simulink model "GVCU_HIL_simscape"  (R2026a)
settings: Solver=ode3  StartTime=0  StopTime=10  FixedStep=0.001
model workspace (MAT data in the model file):
  CANoelibParameters : object (value not decoded)
values from neighbouring files (symbols this model uses):
  acc_pedal_data = pedal_data.accelerator_pedal_position_t0    [Init_Simscape_main.m]
  acc_pedal_time = pedal_data.t0    [Init_Simscape_main.m]
  brk_pedal_data = brake_pedal_data.shared_brakes_drvrBrkPedlPerc_t0    [Init_Simscape_main.m]
  brk_pedal_time = brake_pedal_data.t0    [Init_Simscape_main.m]
  cycle_len = zeros(1, num_cycles)    [Init_Simscape_main.m]
  cycle_speed_matrix = zeros(max_cycle_len, num_cycles)    [Init_Simscape_main.m]
  cycle_time_matrix = zeros(max_cycle_len, num_cycles)    [Init_Simscape_main.m]
  veh_speed_data = speed_data.shared_dynamicsVso_vehVelLgt_t0    [Init_Simscape_main.m]
  veh_speed_time = speed_data.t0    [Init_Simscape_main.m]
undefined symbols (not defined in the file or in its folder): Active, aero, AuxActive, bat, brake, config, environment, FL, FL_prs_voltage, FR, FR_prs_voltage, front, pos, powertrain, rear, RL, RL_prs_voltage, RR, RR_prs_voltage, tir, veh, VGetRawValueFlag, Voltage, VT2816_1_Ch1, VT2816_1_Ch2, VT2816_1_Ch3, VT2816_1_Ch4, VT2816_3_Ch13, VT2816_3_Ch14, VT7101_1_Out2, VTS, X, Y, Z
libraries: sm_lib x358, fl_lib x272, nesl_utility x193, canoelib x127, sdl_lib x36, autolibsharedcoupling x21, autolibcoupling x9, slpidlib x7, simulink x3, autolibshareddiff x3, autolibshared x3, autolibutils x1
(part 17 of 17)

== system GVCU_HIL_simscape/vehicle/powertrain/motor/Subsystem ==
  EM_trq_out : Inport
  Ideal Torque Source1 : fl_lib/Mechanical/Mechanical Sources/Ideal Torque Source
  MRRef1 : fl_lib/Mechanical/Rotational Elements/Mechanical Rotational Reference
  PS Lookup Table (2D)1 : fl_lib/Physical Signals/Lookup Tables/PS Lookup Table (2D)  x1=[-1 powertrain.motor.throttle_bp]  x2=[flip(-powertrain.motor.rpm_bp(2:end)) powertrain.motor.rpm_bp] rad/s  f=[flip(-powertrain.motor.torque_bp(2:end)) -powertrain.motor.torque_bp; flip(powertrain.motor.torque_map(1,2:end)) powertrain.motor.torque_map(1,:); flip(powertrain.motor.torque_map(2,2:end)) powertrain.motor.torque_map(2,:)]  interp_method=simscape.enum.interpolation.linear  extrap_method=simscape.enum.extrapolation.nearest
  Simulink-PS Converter : nesl_utility/Simulink-PS Converter  Commented=on  PhysicalDomain=network_engine_domain  SubClassName=ps_input  LeftPortType=input  RightPortType=output  PseudoPeriodic=off  Frequencies=[]  NoiseDistribution=none  NoiseParameters=[]  Unit=1  AffineConversion=off  FilteringAndDerivatives=provide  SimscapeFilterOrder=1  InputFilterTimeConstant=0.001  UdotUserProvided=0
  throttle : PMIOPort  Side=Left
  omega : PMIOPort  Port=2  Side=Left
  Conn2 : PMIOPort  Port=3  Side=Right
  wires:
  EM_trq_out/1 -> Simulink-PS Converter/1
  connections:
  MRRef1/LConn1 -- Ideal Torque Source1/RConn2
  Ideal Torque Source1/LConn1 -- Conn2/RConn1
  PS Lookup Table (2D)1/LConn2 -- omega/RConn1
  throttle/RConn1 -- PS Lookup Table (2D)1/LConn1
  PS Lookup Table (2D)1/RConn1 -- Ideal Torque Source1/RConn1

== system GVCU_HIL_simscape/vehicle/powertrain/motor/Subsystem3 ==
  Ideal Rotational Motion Sensor : fl_lib/Mechanical/Mechanical Sensors/Ideal Rotational Motion Sensor  reference=foundation.enum.MeasurementReference.difference  acceleration_port=false  velocity_port=true  position_port=false  wrap_angle=false  offset=0 rad
  Ideal Torque Sensor : fl_lib/Mechanical/Mechanical Sensors/Ideal Torque Sensor
  Mechanical Rotational Reference : fl_lib/Mechanical/Rotational Elements/Mechanical Rotational Reference
  PS-Simulink Converter1 : nesl_utility/PS-Simulink Converter  PhysicalDomain=network_engine_domain  SubClassName=ps_output  LeftPortType=input  RightPortType=output  PseudoPeriodic=off  Frequencies=[]  VectorFormat=inherit  Unit=inherit  AffineConversion=off
  PS-Simulink Converter6 : nesl_utility/PS-Simulink Converter  PhysicalDomain=network_engine_domain  SubClassName=ps_output  LeftPortType=input  RightPortType=output  PseudoPeriodic=off  Frequencies=[]  VectorFormat=inherit  Unit=inherit  AffineConversion=off
  in : PMIOPort  Side=Left
  out : PMIOPort  Port=2  Side=Right
  w : Outport
  t : Outport  Port=2
  wires:
  PS-Simulink Converter6/1 -> w/1
  PS-Simulink Converter1/1 -> t/1
  connections:
  Mechanical Rotational Reference/LConn1 -- Ideal Rotational Motion Sensor/RConn1
  PS-Simulink Converter6/LConn1 -- Ideal Rotational Motion Sensor/RConn2
  PS-Simulink Converter1/LConn1 -- Ideal Torque Sensor/RConn2
  in/RConn1 -- Ideal Torque Sensor/LConn1 -- Ideal Rotational Motion Sensor/LConn1
  Ideal Torque Sensor/RConn1 -- out/RConn1

== system GVCU_HIL_simscape/vehicle/powertrain/motor/friction ==
  Ideal Rotational Motion Sensor : fl_lib/Mechanical/Mechanical Sensors/Ideal Rotational Motion Sensor  reference=foundation.enum.MeasurementReference.difference  acceleration_port=false  velocity_port=true  position_port=false  wrap_angle=false  offset=0 rad
  Inertia2 : fl_lib/Mechanical/Rotational Elements/Inertia  inertia=0.05 kg*m^2  num_ports=foundation.enum.numPorts2.one  w_specify=off  w_priority=High  w=0 rad/s  w_nominal_specify=off  w_nominal_value=1  w_nominal_unit=rad/s  t_specify=off  t_priority=None  t=0 N*m  t_nominal_specify=off  t_nominal_value=1  t_nominal_unit=N*m
  Mechanical Rotational Reference : fl_lib/Mechanical/Rotational Elements/Mechanical Rotational Reference
  PS Transfer Function : fl_lib/Physical Signals/Linear Operators/PS Transfer Function  transfer_function_type=foundation.enum.transfer_function_type.lag  T=0.01 s  T1=2 s  T2=1 s  reset_method=foundation.enum.IntegratorResetSpec.None  initial_condition_spec=foundation.enum.IntegratorICSpec.Internal  y0=0 rad/s
  in : PMIOPort  Side=Left
  out : PMIOPort  Port=2  Side=Right
  omega : PMIOPort  Port=3  Side=Right
  connections:
  in/RConn1 -- Inertia2/LConn1 -- Ideal Rotational Motion Sensor/LConn1 -- out/RConn1
  Ideal Rotational Motion Sensor/RConn2 -- PS Transfer Function/LConn1
  Mechanical Rotational Reference/LConn1 -- Ideal Rotational Motion Sensor/RConn1
  omega/RConn1 -- PS Transfer Function/RConn1

== system GVCU_HIL_simscape/vehicle/powertrain/motor/rev limiter ==
  <AccelCmd> : Inport
  PS Constant : fl_lib/Physical Signals/Sources/PS Constant  constant=10000*pi/30
  PS Divide : fl_lib/Physical Signals/Functions/PS Divide
  PS Lookup Table (1D) : fl_lib/Physical Signals/Lookup Tables/PS Lookup Table (1D)  x=[1 1.01] rad/s  f=[1 0]  interp_method=simscape.enum.interpolation.linear  extrap_method=simscape.enum.extrapolation.nearest
  PS Product : fl_lib/Physical Signals/Functions/PS Product
  Simulink-PS Converter : nesl_utility/Simulink-PS Converter  PhysicalDomain=network_engine_domain  SubClassName=ps_input  LeftPortType=input  RightPortType=output  PseudoPeriodic=off  Frequencies=[]  NoiseDistribution=none  NoiseParameters=[]  Unit=1  AffineConversion=off  FilteringAndDerivatives=filter  SimscapeFilterOrder=2  InputFilterTimeConstant=0.001  UdotUserProvided=0
  omega : PMIOPort  Side=Left
  throttle : PMIOPort  Port=2  Side=Right
  wires:
  <AccelCmd>/1 -> Simulink-PS Converter/1
  connections:
  PS Divide/LConn1 -- omega/RConn1
  PS Constant/RConn1 -- PS Divide/LConn2
  PS Divide/RConn1 -- PS Lookup Table (1D)/LConn1
  PS Product/LConn2 -- PS Lookup Table (1D)/RConn1
  Simulink-PS Converter/RConn1 -- PS Product/LConn1
  throttle/RConn1 -- PS Product/RConn1

== system GVCU_HIL_simscape/vehicle/powertrain/side gearbox/Subsystem1 ==
  Ideal Rotational Motion Sensor : fl_lib/Mechanical/Mechanical Sensors/Ideal Rotational Motion Sensor  reference=foundation.enum.MeasurementReference.difference  acceleration_port=false  velocity_port=true  position_port=false  wrap_angle=false  offset=0 rad
  Ideal Torque Sensor : fl_lib/Mechanical/Mechanical Sensors/Ideal Torque Sensor
  Mechanical Rotational Reference : fl_lib/Mechanical/Rotational Elements/Mechanical Rotational Reference
  PS-Simulink Converter1 : nesl_utility/PS-Simulink Converter  PhysicalDomain=network_engine_domain  SubClassName=ps_output  LeftPortType=input  RightPortType=output  PseudoPeriodic=off  Frequencies=[]  VectorFormat=inherit  Unit=inherit  AffineConversion=off
  PS-Simulink Converter6 : nesl_utility/PS-Simulink Converter  PhysicalDomain=network_engine_domain  SubClassName=ps_output  LeftPortType=input  RightPortType=output  PseudoPeriodic=off  Frequencies=[]  VectorFormat=inherit  Unit=inherit  AffineConversion=off
  in : PMIOPort  Side=Left
  out : PMIOPort  Port=2  Side=Right
  w : Outport
  t : Outport  Port=2
  wires:
  PS-Simulink Converter1/1 -> t/1
  PS-Simulink Converter6/1 -> w/1
  connections:
  Ideal Torque Sensor/RConn1 -- out/RConn1
  Ideal Rotational Motion Sensor/LConn1 -- Ideal Torque Sensor/LConn1 -- in/RConn1
  PS-Simulink Converter1/LConn1 -- Ideal Torque Sensor/RConn2
  PS-Simulink Converter6/LConn1 -- Ideal Rotational Motion Sensor/RConn2
  Mechanical Rotational Reference/LConn1 -- Ideal Rotational Motion Sensor/RConn1

== system GVCU_HIL_simscape/vehicle/powertrain/side gearbox/Subsystem3 ==
  Ideal Rotational Motion Sensor : fl_lib/Mechanical/Mechanical Sensors/Ideal Rotational Motion Sensor  reference=foundation.enum.MeasurementReference.difference  acceleration_port=false  velocity_port=true  position_port=false  wrap_angle=false  offset=0 rad
  Ideal Torque Sensor : fl_lib/Mechanical/Mechanical Sensors/Ideal Torque Sensor
  Mechanical Rotational Reference : fl_lib/Mechanical/Rotational Elements/Mechanical Rotational Reference
  PS-Simulink Converter1 : nesl_utility/PS-Simulink Converter  PhysicalDomain=network_engine_domain  SubClassName=ps_output  LeftPortType=input  RightPortType=output  PseudoPeriodic=off  Frequencies=[]  VectorFormat=inherit  Unit=inherit  AffineConversion=off
  PS-Simulink Converter6 : nesl_utility/PS-Simulink Converter  PhysicalDomain=network_engine_domain  SubClassName=ps_output  LeftPortType=input  RightPortType=output  PseudoPeriodic=off  Frequencies=[]  VectorFormat=inherit  Unit=inherit  AffineConversion=off
  in : PMIOPort  Side=Left
  out : PMIOPort  Port=2  Side=Right
  w : Outport
  t : Outport  Port=2
  wires:
  PS-Simulink Converter6/1 -> w/1
  PS-Simulink Converter1/1 -> t/1
  connections:
  Mechanical Rotational Reference/LConn1 -- Ideal Rotational Motion Sensor/RConn1
  PS-Simulink Converter6/LConn1 -- Ideal Rotational Motion Sensor/RConn2
  PS-Simulink Converter1/LConn1 -- Ideal Torque Sensor/RConn2
  in/RConn1 -- Ideal Torque Sensor/LConn1 -- Ideal Rotational Motion Sensor/LConn1
  Ideal Torque Sensor/RConn1 -- out/RConn1

== system GVCU_HIL_simscape/vehicle/powertrain/transmission/Subsystem3 ==
  Ideal Rotational Motion Sensor : fl_lib/Mechanical/Mechanical Sensors/Ideal Rotational Motion Sensor  reference=foundation.enum.MeasurementReference.difference  acceleration_port=false  velocity_port=true  position_port=false  wrap_angle=false  offset=0 rad
  Ideal Torque Sensor : fl_lib/Mechanical/Mechanical Sensors/Ideal Torque Sensor
  Mechanical Rotational Reference : fl_lib/Mechanical/Rotational Elements/Mechanical Rotational Reference
  PS-Simulink Converter1 : nesl_utility/PS-Simulink Converter  PhysicalDomain=network_engine_domain  SubClassName=ps_output  LeftPortType=input  RightPortType=output  PseudoPeriodic=off  Frequencies=[]  VectorFormat=inherit  Unit=inherit  AffineConversion=off
  PS-Simulink Converter6 : nesl_utility/PS-Simulink Converter  PhysicalDomain=network_engine_domain  SubClassName=ps_output  LeftPortType=input  RightPortType=output  PseudoPeriodic=off  Frequencies=[]  VectorFormat=inherit  Unit=inherit  AffineConversion=off
  in : PMIOPort  Side=Left
  out : PMIOPort  Port=2  Side=Right
  w : Outport
  t : Outport  Port=2
  wires:
  PS-Simulink Converter6/1 -> w/1
  PS-Simulink Converter1/1 -> t/1
  connections:
  Mechanical Rotational Reference/LConn1 -- Ideal Rotational Motion Sensor/RConn1
  PS-Simulink Converter6/LConn1 -- Ideal Rotational Motion Sensor/RConn2
  PS-Simulink Converter1/LConn1 -- Ideal Torque Sensor/RConn2
  in/RConn1 -- Ideal Torque Sensor/LConn1 -- Ideal Rotational Motion Sensor/LConn1
  Ideal Torque Sensor/RConn1 -- out/RConn1

== system GVCU_HIL_simscape/vehicle/powertrain/transmission/gear selector ==
  In1 : Inport
  Clutches Gear 1 : Constant  Value=[0 0 0 0 0 0 0 0 0]  SampleTime=0
  Clutches Gear 10 : Constant  Value=[0 0 0 0 0 0 0 1 0]  SampleTime=0
  Clutches Gear 11 : Constant  Value=[0 0 0 0 0 0 0 0 1]  SampleTime=0
  Clutches Gear 2 : Constant  Value=[1 0 0 0 0 0 0 0 0]  SampleTime=0
  Clutches Gear 3 : Constant  Value=[0 1 0 0 0 0 0 0 0]  SampleTime=0
  Clutches Gear 4 : Constant  Value=[0 0 0 0 0 0 0 0 0]  SampleTime=0
  Clutches Gear 5 : Constant  Value=[0 0 1 0 0 0 0 0 0]  SampleTime=0
  Clutches Gear 6 : Constant  Value=[0 0 0 1 0 0 0 0 0]  SampleTime=0
  Clutches Gear 7 : Constant  Value=[0 0 0 0 1 0 0 0 0]  SampleTime=0
  Clutches Gear 8 : Constant  Value=[0 0 0 0 0 1 0 0 0]  SampleTime=0
  Clutches Gear 9 : Constant  Value=[0 0 0 0 0 0 1 0 0]  SampleTime=0
  Demux : Demux  Outputs=9
  Multiport Switch : MultiPortSwitch  DataPortOrder=Specify indices  DataPortIndices={-1,0,1,2,3,4,5,6,7,8,9}  SaturateOnIntegerOverflow=off  InputSameDT=off
  Simulink-PS Converter{1..9} (9 alike) : nesl_utility/Simulink-PS Converter  PhysicalDomain=network_engine_domain  SubClassName=ps_input  LeftPortType=input  RightPortType=output  PseudoPeriodic=off  Frequencies=[]  NoiseDistribution=none  NoiseParameters=[]  Unit=1  AffineConversion=off  FilteringAndDerivatives=provide  SimscapeFilterOrder=1  InputFilterTimeConstant=0.001  UdotUserProvided=0
  1 : PMIOPort  Side=Right
  2 : PMIOPort  Port=2  Side=Right
  3 : PMIOPort  Port=3  Side=Right
  4 : PMIOPort  Port=4  Side=Right
  5 : PMIOPort  Port=5  Side=Right
  6 : PMIOPort  Port=6  Side=Right
  7 : PMIOPort  Port=7  Side=Right
  8 : PMIOPort  Port=8  Side=Right
  9 : PMIOPort  Port=9  Side=Right
  wires:
  Demux/5 -> Simulink-PS Converter4/1
  Clutches Gear 3/1 -> Multiport Switch/5
  Demux/4 -> Simulink-PS Converter3/1
  Clutches Gear 8/1 -> Multiport Switch/9
  Clutches Gear 5/1 -> Multiport Switch/6
  Clutches Gear 7/1 -> Multiport Switch/8
  Clutches Gear 10/1 -> Multiport Switch/11
  Clutches Gear 6/1 -> Multiport Switch/7
  Clutches Gear 11/1 -> Multiport Switch/12
  Clutches Gear 1/1 -> Multiport Switch/3
  Clutches Gear 2/1 -> Multiport Switch/4
  Demux/3 -> Simulink-PS Converter7/1
  Demux/7 -> Simulink-PS Converter6/1
  Demux/2 -> Simulink-PS Converter1/1
  Demux/1 -> Simulink-PS Converter2/1
  Clutches Gear 4/1 -> Multiport Switch/2
  Demux/8 -> Simulink-PS Converter8/1
  Demux/9 -> Simulink-PS Converter9/1
  Clutches Gear 9/1 -> Multiport Switch/10
  Multiport Switch/1 -> Demux/1
  Demux/6 -> Simulink-PS Converter5/1
  In1/1 -> Multiport Switch/1
  connections:
  Simulink-PS Converter2/RConn1 -- 1/RConn1
  3/RConn1 -- Simulink-PS Converter7/RConn1
  6/RConn1 -- Simulink-PS Converter5/RConn1
  4/RConn1 -- Simulink-PS Converter3/RConn1
  7/RConn1 -- Simulink-PS Converter6/RConn1
  5/RConn1 -- Simulink-PS Converter4/RConn1
  9/RConn1 -- Simulink-PS Converter9/RConn1
  8/RConn1 -- Simulink-PS Converter8/RConn1
  2/RConn1 -- Simulink-PS Converter1/RConn1

== system GVCU_HIL_simscape/vehicle/multibody/chassis/Subsystem/Subsystem ==
  1 : Inport
  2 : Inport  Port=2
  Add : Sum  Inputs=+++
  Constant : Constant  Value=eps
  Divide : Product  Inputs=*/
  Out1 : Outport
  wires:
  Divide/1 -> Out1/1
  Add/1 -> Divide/2
  2/1 -> Add/2
  1/1 -> Divide/1, Add/1
  Constant/1 -> Add/3

== system GVCU_HIL_simscape/vehicle/multibody/chassis/Subsystem/drag force ==
  PS Constant : fl_lib/Physical Signals/Sources/PS Constant  constant=1/2
  PS Constant1 : fl_lib/Physical Signals/Sources/PS Constant  constant=1.225 kg/m^3
  PS Constant2 : fl_lib/Physical Signals/Sources/PS Constant  constant=aero.A m^2
  PS Gain : fl_lib/Physical Signals/Functions/PS Gain  gain=-1
  PS Lookup Table (2D) : fl_lib/Physical Signals/Lookup Tables/PS Lookup Table (2D)  x1=aero.FRH m  x2=aero.RRH m  f=aero.Cd  interp_method=simscape.enum.interpolation.linear  extrap_method=simscape.enum.extrapolation.linear
  PS Product{,1..5} (6 alike) : fl_lib/Physical Signals/Functions/PS Product
  PS Sign : fl_lib/Physical Signals/Nonlinear Operators/PS Sign
  vx : PMIOPort  Side=Left
  fx : PMIOPort  Port=2  Side=Right
  frh : PMIOPort  Port=3  Side=Left
  rrh : PMIOPort  Port=4  Side=Left
  connections:
  vx/RConn1 -- PS Sign/LConn1 -- PS Product4/LConn2 -- PS Product4/LConn1
  PS Lookup Table (2D)/RConn1 -- PS Product/LConn2
  PS Product2/RConn1 -- PS Product1/LConn1
  PS Product3/RConn1 -- PS Product2/LConn1
  PS Constant1/RConn1 -- PS Product2/LConn2
  PS Constant2/RConn1 -- PS Product1/LConn2
  PS Product3/LConn2 -- PS Constant/RConn1
  PS Product4/RConn1 -- PS Product5/LConn1
  PS Product1/RConn1 -- PS Product/LConn1
  PS Gain/LConn1 -- PS Product/RConn1
  PS Product5/RConn1 -- PS Product3/LConn1
  PS Sign/RConn1 -- PS Product5/LConn2
  fx/RConn1 -- PS Gain/RConn1
  frh/RConn1 -- PS Lookup Table (2D)/LConn1
  rrh/RConn1 -- PS Lookup Table (2D)/LConn2

== system GVCU_HIL_simscape/vehicle/multibody/chassis/Subsystem/front downforce ==
  PS Constant : fl_lib/Physical Signals/Sources/PS Constant  constant=1/2
  PS Constant1 : fl_lib/Physical Signals/Sources/PS Constant  constant=1.225 kg/m^3
  PS Constant2 : fl_lib/Physical Signals/Sources/PS Constant  constant=aero.A m^2
  PS Lookup Table (2D) : fl_lib/Physical Signals/Lookup Tables/PS Lookup Table (2D)  x1=aero.FRH m  x2=aero.RRH m  f=aero.Clf  interp_method=simscape.enum.interpolation.linear  extrap_method=simscape.enum.extrapolation.linear
  PS Product{,1..4} (5 alike) : fl_lib/Physical Signals/Functions/PS Product
  vx : PMIOPort  Side=Left
  frh : PMIOPort  Port=2  Side=Left
  rrh : PMIOPort  Port=3  Side=Left
  fz : PMIOPort  Port=4  Side=Right
  connections:
  PS Product4/LConn2 -- PS Product4/LConn1 -- vx/RConn1
  PS Product2/LConn1 -- PS Product3/RConn1
  PS Product3/LConn2 -- PS Constant/RConn1
  PS Product2/RConn1 -- PS Product1/LConn1
  PS Product/LConn1 -- PS Product1/RConn1
  fz/RConn1 -- PS Product/RConn1
  PS Constant1/RConn1 -- PS Product2/LConn2
  PS Lookup Table (2D)/RConn1 -- PS Product/LConn2
  PS Product4/RConn1 -- PS Product3/LConn1
  PS Constant2/RConn1 -- PS Product1/LConn2
  PS Lookup Table (2D)/LConn1 -- frh/RConn1
  rrh/RConn1 -- PS Lookup Table (2D)/LConn2

== system GVCU_HIL_simscape/vehicle/multibody/chassis/Subsystem/rear downforce ==
  PS Constant : fl_lib/Physical Signals/Sources/PS Constant  constant=1/2
  PS Constant1 : fl_lib/Physical Signals/Sources/PS Constant  constant=1.225 kg/m^3
  PS Constant2 : fl_lib/Physical Signals/Sources/PS Constant  constant=aero.A m^2
  PS Lookup Table (2D) : fl_lib/Physical Signals/Lookup Tables/PS Lookup Table (2D)  x1=aero.FRH m  x2=aero.RRH m  f=aero.Clr  interp_method=simscape.enum.interpolation.linear  extrap_method=simscape.enum.extrapolation.linear
  PS Product{,1..4} (5 alike) : fl_lib/Physical Signals/Functions/PS Product
  vx : PMIOPort  Side=Left
  fz : PMIOPort  Port=2  Side=Right
  frh : PMIOPort  Port=3  Side=Left
  rrh : PMIOPort  Port=4  Side=Left
  connections:
  vx/RConn1 -- PS Product4/LConn2 -- PS Product4/LConn1
  PS Product3/LConn2 -- PS Constant/RConn1
  fz/RConn1 -- PS Product/RConn1
  PS Product4/RConn1 -- PS Product3/LConn1
  PS Lookup Table (2D)/RConn1 -- PS Product/LConn2
  PS Product/LConn1 -- PS Product1/RConn1
  PS Constant2/RConn1 -- PS Product1/LConn2
  PS Constant1/RConn1 -- PS Product2/LConn2
  PS Product2/RConn1 -- PS Product1/LConn1
  PS Product2/LConn1 -- PS Product3/RConn1
  frh/RConn1 -- PS Lookup Table (2D)/LConn1
  rrh/RConn1 -- PS Lookup Table (2D)/LConn2

== system GVCU_HIL_simscape/vehicle/multibody/chassis/Subsystem1/Subsystem ==
  note: not possible to handle pitch +/- 90 degrees according to source
  R : Inport
  Asin : Trigonometry  Operator=asin
  Atan1 : Trigonometry  Operator=atan2
  Atan2 : Trigonometry  Operator=atan2
  Demux : Demux  Outputs=2
  Demux1 : Demux  Outputs=2
  Gain : Gain  Gain=-1
  "R(3, 1)" : Selector  NumberOfDimensions=2  InputPortWidth=3  IndexOptions=Index vector (dialog),Index vector (dialog)  Indices=3,1  OutputSizes=1,1
  "R(3, 2:3)" : Selector  NumberOfDimensions=2  InputPortWidth=3  IndexOptions=Index vector (dialog),Index vector (dialog)  Indices=3,[2 3]  OutputSizes=1,1
  "R([2 1], 1)" : Selector  NumberOfDimensions=2  InputPortWidth=3  IndexOptions=Index vector (dialog),Index vector (dialog)  Indices=[2 1],1  OutputSizes=1,1
  Reshape : Reshape
  Reshape1 : Reshape
  Reshape2 : Reshape  OutputDimensionality=Customize  OutputDimensions=1
  roll : Outport  VectorParamsAs1DForOutWhenUnconnected=off
  pitch : Outport  Port=2  VectorParamsAs1DForOutWhenUnconnected=off
  yaw : Outport  Port=3  VectorParamsAs1DForOutWhenUnconnected=off
  wires:
  Demux/1 -> Atan2/1
  Atan2/1 -> Reshape2/1
  Demux1/1 -> Atan1/1
  Demux1/2 -> Atan1/2
  Gain/1 -> Asin/1
  Demux/2 -> Atan2/2
  "R([2 1], 1)"/1 -> Demux1/1
  Asin/1 -> Reshape1/1
  "R(3, 2:3)"/1 -> Demux/1
  Reshape/1 -> yaw/1
  Atan1/1 -> Reshape/1
  R/1 -> "R([2 1], 1)"/1, "R(3, 2:3)"/1, "R(3, 1)"/1
  Reshape2/1 -> roll/1
  Reshape1/1 -> pitch/1
  "R(3, 1)"/1 -> Gain/1

== system GVCU_HIL_simscape/vehicle/multibody/chassis/local coordinates/Subsystem ==
  In1 : Inport
  Asin : Trigonometry  Operator=asin
  Cos : Trigonometry  Operator=cos
  Demux : Demux  Outputs=3
  Derivative : Derivative
  Derivative1 : Derivative
  Divide : Product  Inputs=*/
  Divide1 : Product  Inputs=*/
  Gain : Gain  Gain=-1
  Mux : Mux  Inputs=2
  Selector : Selector  NumberOfDimensions=2  InputPortWidth=3  IndexOptions=Index vector (dialog),Index vector (dialog)  Indices=[1 2 3],2  OutputSizes=1,1
  Selector1 : Selector  NumberOfDimensions=2  InputPortWidth=3  IndexOptions=Index vector (dialog),Index vector (dialog)  Indices=[1 2 3],1  OutputSizes=1,1
  Selector2 : Selector  InputPortWidth=3  IndexOptions=Index vector (dialog)  Indices=[3]  OutputSizes=1
  Trigonometric Function1 : Trigonometry  Operator=atan2
  magnitude : Fcn  Expr=sqrt(u(1)*u(1)+u(2)*u(2))
  magnitude1 : Fcn  Expr=sqrt(u(1)*u(1)+u(2)*u(2)+u(3)*u(3))
  aRoll : Outport
  aPitch : Outport  Port=2
  nRoll : Outport  Port=3
  nPitch : Outport  Port=4
  wires:
  Derivative1/1 -> nRoll/1
  Derivative/1 -> nPitch/1
  Gain/1 -> aPitch/1, Derivative/1
  Selector2/1 -> Divide/1
  Asin/1 -> Gain/1
  magnitude1/1 -> Divide1/2
  Divide/1 -> Divide1/1
  Selector1/1 -> magnitude1/1, Selector2/1
  Cos/1 -> Divide/2
  Trigonometric Function1/1 -> Cos/1, aRoll/1, Derivative1/1
  Divide1/1 -> Asin/1
  Selector/1 -> Demux/1
  Demux/3 -> Trigonometric Function1/1
  Mux/1 -> magnitude/1
  Demux/1 -> Mux/1
  magnitude/1 -> Trigonometric Function1/2
  Demux/2 -> Mux/2
  In1/1 -> Selector/1, Selector1/1

== matlab function GVCU_HIL_simscape/Clutch handling/Offset_substraction/MATLAB Function ==
  data: drvMode input; y output; pPa input
function y = fcn(drvMode, pPa)
% drvMode : drive mode input
% pPa     : measured pressure input in Pa
% y       : pressure output with learned offset removed, in Pa

persistent prevDrvMode state timer sumP sampleCount offset

if isempty(prevDrvMode)
    prevDrvMode = drvMode;
    state = uint8(0);      % 0=idle, 1=wait, 2=average, 3=hold
    timer = 0.0;
    sumP = 0.0;
    sampleCount = uint32(0);
    offset = 0.0;
end

T = 0.0002;          % sample time [s]
WAIT_TIME = 0.5;     % wait time after drvMode becomes 1 [s]
AVG_TIME  = 0.2;     % averaging time [s]
ONE_BAR_PA = 1e5;    % 1 bar in Pa

% Trigger when drvMode becomes 1, regardless of previous value
if (prevDrvMode ~= 1) && (drvMode == 1)
    state = uint8(1);
    timer = 0.0;
    sumP = 0.0;
    sampleCount = uint32(0);
end

switch state
    case 0
        % Idle state

    case 1
        % Wait for 0.5 s
        timer = timer + T;
        if timer >= WAIT_TIME
            state = uint8(2);
            timer = 0.0;
            sumP = 0.0;
            sampleCount = uint32(0);
        end

    case 2
        % Average pressure for 0.2 s
        timer = timer + T;
        sumP = sumP + pPa;
        sampleCount = sampleCount + 1;

        if timer >= AVG_TIME
            if sampleCount > 0
                offset = sumP / double(sampleCount) - ONE_BAR_PA;
            else
                offset = 0.0;
            end
            state = uint8(3);
        end

    case 3
        % Hold learned offset
end

% Output compensated pressure
y = pPa - offset;

prevDrvMode = drvMode;

== matlab function GVCU_HIL_simscape/Powertrain (EV)/PID Speed Ctrl Mode/MATLAB Function1 ==
  settings: updateMethod=DISCRETE
  data: spdErr_rads input; trq_cmd output; trq_fwd input; trq_act input; lim_pos input; lim_neg input; reset input
function trq_cmd = speedPID(spdErr_rads, trq_fwd, trq_act, lim_pos, lim_neg, reset)
%#codegen
% Speed PID + feedforward, output clamped.
% Replicates inverter torque_handler.c trqHandlerSpeedCtrl()
%
% Inputs:
%   spdErr_rads  [rad/s]   speed error (spd_req - spd_fb), computed externally
%   trq_fwd      [Nm]      feedforward torque = GVCU torque request (added internally)
%   trq_act      [Nm]      actual motor torque feedback (e.g. EM_trq from motor model)
%   lim_pos      [Nm]      upper output clamp
%   lim_neg      [Nm]      lower output clamp
%   reset                  from spdCtrlReset block (>0.5 = active)
%
% Output:
%   trq_cmd  [Nm]      clamped torque command (PID + feedforward)
%
% Gains (caldata.c index 0, RPM-based, Ts=500us):
%   kp=2.5, ki=0.004, kaw=0.0035, kd=0

persistent intgl trqReqPrev

if isempty(intgl)
    intgl      = 0;
    trqReqPrev = 0;
end

Ts      = 0.0002;       % actual Simulink step size
Ts_inv  = 0.0005;       % inverter design step size
scale   = Ts / Ts_inv;  % = 0.4

% values from Set 3 
kp  = 2; %0.78;
ki  = 0.035 * scale;    % = 0.0016
kaw = 0.005 * scale;   % = 0.0014

if reset > 0.5
    intgl      = 0;
    trqReqPrev = 0;
    trq_cmd    = 0;
    return;
end

% Speed error in RPM (matches inverter: spdErr = spdReq - ctrlOutSpeed)
spdErr = spdErr_rads * (60 / (2*pi));

% Integrator update with anti-windup
% Matches inverter: spdIntgl += ki*spdErr + kaw*(trqAct - trqReq_prev_unclamped)
intgl = intgl + ki * spdErr + kaw * (trq_act - trqReqPrev);

% Unclamped total output (PID + feedforward)
trq_req_unc = kp * spdErr + intgl + trq_fwd;

% Clamp output
trq_cmd = max(lim_neg, min(lim_pos, trq_req_unc));

% Store unclamped total for next step's anti-windup
trqReqPrev = trq_cmd;

== matlab function GVCU_HIL_simscape/vehicle/powertrain/brakes/ABS/MATLAB Function ==
  data: decel input; ABSCmd input; decel_FL output; FL input; FR input; RL input; RR input; decel_FR output; decel_RL output; decel_RR output
function [decel_FL,decel_FR,decel_RL,decel_RR] = fcn(decel,ABSCmd,FL,FR,RL,RR)

if ABSCmd == 1
    decel_FL = decel*FL;
    decel_FR = decel*FR;
    decel_RL = decel*RL;
    decel_RR = decel*RR;
else
    decel_FL = decel;
    decel_FR = decel;
    decel_RL = decel;
    decel_RR = decel;
end

== matlab function GVCU_HIL_simscape/vehicle/powertrain/engine/TC/MATLAB Function ==
  data: accel input; accel_out output; TC input; slip_error input; TCCmd input
function accel_out = fcn(accel,TC,slip_error,TCCmd)

if TCCmd == 1 && slip_error > 0.1
    accel_out = accel*TC;
else
    accel_out = accel;
end

== matlab function GVCU_HIL_simscape/Driver/brake balance/brake balance ==
  data: right1 input; left1 input; BrakeBalCmd output; right2 input; left2 input; BrakeBal_max input; BrakeBal_min input; BrakeBal_default input; BrakeBal_act input
function BrakeBalCmd = fcn(right1,left1,right2,left2,BrakeBal_max,BrakeBal_min,BrakeBal_default,BrakeBal_act)

if BrakeBal_act == 0
    BrakeBal_act = BrakeBal_default;
end

if right1 == 1 && right2 == 0 && BrakeBal_act <= BrakeBal_max
    BrakeBal_act = BrakeBal_act + 0.01;
elseif left1 == 1 && left2 == 0 && BrakeBal_act >= BrakeBal_min
    BrakeBal_act = BrakeBal_act - 0.01;
end

BrakeBalCmd = BrakeBal_act;

== matlab function GVCU_HIL_simscape/Powertrain (EV)/PID Speed Controller/MATLAB Function ==
  settings: updateMethod=DISCRETE
  data: EM_Spd input; reset_out output; speed_req input; t input
function reset_out = spdCtrlReset(EM_Spd, speed_req, t)
% Resets PID integrator when both speeds are below threshold for 500ms.
% Matches real inverter: cInvStopSpeed = 20 RPM, SPD_CTRL_RESET_DELAY = 500ms
% Input t: simulation time from Clock block [s]

persistent stop_ts fired

if isempty(stop_ts)
    stop_ts = 0;
    fired   = false;
end

SPD_THRESHOLD  = 2.094;  % 20 RPM in rad/s  (= cInvStopSpeed)
RESET_DELAY_S  = 0.5;    % 500ms in s       (= SPD_CTRL_RESET_DELAY)

if (abs(EM_Spd) < SPD_THRESHOLD) && (abs(speed_req) < SPD_THRESHOLD)
    if stop_ts == 0
        stop_ts = t;     % Start timer: record entry time
    end

    if ((t - stop_ts) >= RESET_DELAY_S) && (~fired)
        reset_out = 1.0; % Rising edge -> reset PID integrator
        fired     = true;
    else
        reset_out = 0.0;
    end
else
    stop_ts   = 0;       % Reset timer
    fired     = false;   % Allow trigger again next standstill
    reset_out = 0.0;
end

== matlab function GVCU_HIL_simscape/Driver/gear/MATLAB Function ==
  settings: updateMethod=DISCRETE
  data: nEngine input; GearCmd output; ax input; gear_max input; nEngine_max input; nEngine_min input; t input; shift_delay input; gear_act input
function GearCmd = fcn(nEngine,ax,gear_max,nEngine_max,nEngine_min,t,shift_delay,gear_act)

if gear_act == 0
    gear_act = 1;
end

persistent last_time

if isempty(last_time)
    last_time = -inf;
end

if t - last_time >= shift_delay
    if nEngine > nEngine_max*pi/30 && gear_act < gear_max
        gear_act = gear_act + 1;
    end
    
    if nEngine < nEngine_min*pi/30 && gear_act > 1 && ax < 0
        gear_act = gear_act - 1;
    end
    last_time = t;
end

GearCmd = gear_act;

== matlab function GVCU_HIL_simscape/Inverter/INV ==
  data: inv_st_prev input; inv_st output; inv_ena_req input; motor_ena_req input; inv_shutdown_req input
function inv_st = fcn(inv_st_prev, inv_ena_req, motor_ena_req, inv_shutdown_req)
	switch inv_st_prev
		case 0
			if (1 == inv_ena_req)
				inv_st_local = 1;
			else
				inv_st_local = 0;
			end
		case 1
			if (1 == inv_ena_req)
				inv_st_local = 2;
			else
				inv_st_local = 0;
			end	
		case 2
			if (1 == inv_ena_req)
				inv_st_local = 3;
			else
				inv_st_local = 0;
			end
		case 3
			if ((1 == inv_ena_req) && (1 == motor_ena_req))
				inv_st_local = 4;
			else
				inv_st_local = 3;
			end
		case 4
			if ((1 ~= inv_ena_req) || (1 ~= motor_ena_req) || (1 == inv_shutdown_req))
				inv_st_local = 0;
			else
				inv_st_local = 4;
			end
		case 5
			inv_st_local = 0;
		case 6
			inv_st_local = 0;
		otherwise
			inv_st_local = 0;
	end
	inv_st = inv_st_local;
 
end

== matlab function GVCU_HIL_simscape/GVCU - HiL/BMS ==
  data: bms_st_prev input; pwr_st input; bms_st output; hyb_st input
function bms_st = fcn(bms_st_prev, pwr_st, hyb_st)
	switch bms_st_prev
		case 0
			bms_st_local = 5;
		case 1
			if (7 ~= pwr_st)
				bms_st_local = 5;
            elseif (4 == hyb_st)
				bms_st_local = 3;
			else
				bms_st_local = 1;
			end	
		case 2
			bms_st_local = 5;
		case 3
			if (7 ~= pwr_st)
				bms_st_local = 5;
			else
				bms_st_local = 3;
			end
		case 4
			bms_st_local = 5;
		case 5
			if (7 == pwr_st)
				bms_st_local = 3;
			else
				bms_st_local = 5;
			end
		case 6
			bms_st_local = 5;
		otherwise
			bms_st_local = 5;
	end
    bms_st = bms_st_local;
end

== matlab function GVCU_HIL_simscape/Wheel_rates/MATLAB Function2 ==
  data: wheel_rate input; wheel_direction output
function wheel_direction = wheel_direction(wheel_rate)

STATIONARY_THD = 0.01; % rad/s
 
if abs(wheel_rate) <= STATIONARY_THD

    wheel_direction = 2; % STATIONARY

elseif wheel_rate > STATIONARY_THD

    wheel_direction = 3; % FORWARD

elseif wheel_rate < -STATIONARY_THD

    wheel_direction = 4; % REARWARD

else

    wheel_direction = 0; % UNKNOWN (NaN)

end

== matlab function GVCU_HIL_simscape/Driver/MATLAB Function ==
  settings: updateMethod=DISCRETE
  data: t_sim input; input_mode input; t_spd input; spd_data input; cycle_idx input; cycle_time_matrix input; cycle_speed_matrix input; cycle_len input; vel_ref input; vel_out output; cycle_time_remaining output; cycle_finished output
function [vel_out, cycle_time_remaining, cycle_finished] = fcn(t_sim, input_mode, t_spd, spd_data, ...
                                                              cycle_idx, cycle_time_matrix, cycle_speed_matrix, cycle_len, vel_ref)

persistent t_mode_start last_mode last_cycle;

if isempty(t_mode_start)
    t_mode_start = -1;
    last_mode    = 0;
    last_cycle   = 0;
end

% Default: WLTC3b
default_cycle_idx = 4;

% Safe cycle index
idx = round(cycle_idx);

if isnan(idx) || idx < 1 || idx > size(cycle_time_matrix, 2)
    idx = default_cycle_idx;
end

% Restart timing when mode changes to replay modes
if (input_mode == 2 || input_mode == 3) && last_mode ~= input_mode
    t_mode_start = t_sim;
end

% Restart drive cycle when selected cycle changes while input_mode == 3
if input_mode == 3 && last_cycle ~= idx
    t_mode_start = t_sim;
end

last_mode  = input_mode;
last_cycle = idx;

% Default outputs
vel_out              = vel_ref;
cycle_time_remaining = 0;
cycle_finished       = 0;

if input_mode == 2 && t_mode_start >= 0

    % Recorded speed replay
    t_rel = t_sim - t_mode_start;
    t_rel = min(t_rel, t_spd(end));

    vel_out = interp1(t_spd, spd_data, t_rel, 'linear', spd_data(end));

elseif input_mode == 3 && t_mode_start >= 0

    % Drive cycle replay
    n = int32(cycle_len(idx));

    cycle_end_time = cycle_time_matrix(n, idx);

    t_rel = t_sim - t_mode_start;

    % Remaining time of selected cycle
    cycle_time_remaining = max(cycle_end_time - t_rel, 0);

    if t_rel >= cycle_end_time
        cycle_finished = 1;
        t_rel = cycle_end_time;
    end

    cycle_time  = cycle_time_matrix(1:n, idx);
    cycle_speed = cycle_speed_matrix(1:n, idx);

    vel_out = interp1(cycle_time, cycle_speed, t_rel, 'linear', cycle_speed(end));

end

== matlab function GVCU_HIL_simscape/Driver/Drive mode/MATLAB Function2 ==
  settings: updateMethod=DISCRETE
  data: RefVel input; RefVel output; trans_park_neutral input; ign output; brake_switch output; btn_paddle_ri output; btn_paddle_le output; trans_neutral_drive input; trans_park_drive input
function [RefVel, ign, brake_switch, btn_paddle_ri, btn_paddle_le] = update_drv_st(RefVel, trans_park_neutral, trans_neutral_drive, trans_park_drive)
persistent main_state sub_state t_start
persistent brake_switch_internal
persistent btn_paddle_ri_internal btn_paddle_le_internal
persistent prev_trans_park_neutral prev_trans_neutral_drive prev_trans_park_drive
persistent pending_park_neutral pending_neutral_drive pending_park_drive

% main_state:
% 0 = idle
% 1 = Park -> Neutral
% 2 = Neutral -> Drive
% 3 = Park -> Drive
%
% signal convention:
% brake_switch: 1 = released, 2 = pressed
% btn_paddle_ri: 1 = released, 2 = pressed
% btn_paddle_le: 1 = released, 2 = pressed

if isempty(main_state)
    main_state = 0;
    sub_state = 0;
    t_start = tic;

    brake_switch_internal = 1;
    btn_paddle_ri_internal = 1;
    btn_paddle_le_internal = 1;

    prev_trans_park_neutral = 0;
    prev_trans_neutral_drive = 0;
    prev_trans_park_drive = 0;

    pending_park_neutral = 0;
    pending_neutral_drive = 0;
    pending_park_drive = 0;
end

ign = 7;
refVelInp = RefVel;

% Capture button rising edges and store as one-shot pending requests.
if trans_park_neutral && ~prev_trans_park_neutral
    pending_park_neutral = 1;
end
if trans_neutral_drive && ~prev_trans_neutral_drive
    pending_neutral_drive = 1;
end
if trans_park_drive && ~prev_trans_park_drive
    pending_park_drive = 1;
end

prev_trans_park_neutral = trans_park_neutral;
prev_trans_neutral_drive = trans_neutral_drive;
prev_trans_park_drive = trans_park_drive;

% Only start a new transition when no other transition is active
if main_state == 0
    if pending_park_drive
        main_state = 3;
        sub_state = 0;
        t_start = tic;
        pending_park_drive = 0;

    elseif pending_park_neutral
        main_state = 1;
        sub_state = 0;
        t_start = tic;
        pending_park_neutral = 0;

    elseif pending_neutral_drive
        main_state = 2;
        sub_state = 0;
        t_start = tic;
        pending_neutral_drive = 0;
    end
end

switch main_state
    case 0
        % Idle:
        % keep RefVel input
        % release buttons and brake
        RefVel = refVelInp;
        brake_switch_internal = 1;
        btn_paddle_ri_internal = 1;
        btn_paddle_le_internal = 1;

    case 1
        % Park -> Neutral
        % RefVel forced to zero during transition
        RefVel = 0;

        switch sub_state
            case 0
                % Press brake first
                brake_switch_internal = 2;
                btn_paddle_ri_internal = 1;
                btn_paddle_le_internal = 1;

                sub_state = 1;
                t_start = tic;

            case 1
                % Press both paddles for 1 second
                brake_switch_internal = 2;
                btn_paddle_ri_internal = 2;
                btn_paddle_le_internal = 2;

                if toc(t_start) >= 1.0
                    sub_state = 2;
                    t_start = tic;
                end

            case 2
                % Release both paddles, keep brake pressed
                brake_switch_internal = 2;
                btn_paddle_ri_internal = 1;
                btn_paddle_le_internal = 1;

                if toc(t_start) >= 0.2
                    sub_state = 3;
                end

            case 3
                % Finish in Neutral, then return to idle
                brake_switch_internal = 1;
                btn_paddle_ri_internal = 1;
                btn_paddle_le_internal = 1;

                main_state = 0;
                sub_state = 0;
        end

    case 2
        % Neutral -> Drive
        % RefVel forced to zero during transition
        RefVel = 0;

        switch sub_state
            case 0
                % Press brake first
                brake_switch_internal = 2;
                btn_paddle_ri_internal = 1;
                btn_paddle_le_internal = 1;

                sub_state = 1;
                t_start = tic;

            case 1
                % Press right paddle for 1 second
                brake_switch_internal = 2;
                btn_paddle_ri_internal = 2;
                btn_paddle_le_internal = 1;

                if toc(t_start) >= 1.0
                    sub_state = 2;
                    t_start = tic;
                end

            case 2
                % Release right paddle, keep brake pressed
                brake_switch_internal = 2;
                btn_paddle_ri_internal = 1;
                btn_paddle_le_internal = 1;

                if toc(t_start) >= 0.2
                    sub_state = 3;
                end

            case 3
                % Release brake after paddle release
                brake_switch_internal = 1;
                btn_paddle_ri_internal = 1;
                btn_paddle_le_internal = 1;

                main_state = 0;
                sub_state = 0;
        end

    case 3
        % Park -> Drive
        % RefVel forced to zero during transition
        RefVel = 0;

        switch sub_state
            case 0
                % Press brake first
                brake_switch_internal = 2;
                btn_paddle_ri_internal = 1;
                btn_paddle_le_internal = 1;

                sub_state = 1;
                t_start = tic;

            case 1
                % Press both paddles for 1 second
                brake_switch_internal = 2;
                btn_paddle_ri_internal = 2;
                btn_paddle_le_internal = 2;

                if toc(t_start) >= 1.0
                    sub_state = 2;
                    t_start = tic;
                end

            case 2
                % Release both paddles -> Neutral, keep brake pressed
                brake_switch_internal = 2;
                btn_paddle_ri_internal = 1;
                btn_paddle_le_internal = 1;

                if toc(t_start) >= 0.2
                    sub_state = 3;
                    t_start = tic;
                end

            case 3
                % Press right paddle for 1 second
                brake_switch_internal = 2;
                btn_paddle_ri_internal = 2;
                btn_paddle_le_internal = 1;

                if toc(t_start) >= 1.0
                    sub_state = 4;
                    t_start = tic;
                end

            case 4
                % Release right paddle -> Drive, keep brake pressed
                brake_switch_internal = 2;
                btn_paddle_ri_internal = 1;
                btn_paddle_le_internal = 1;

                if toc(t_start) >= 0.2
                    sub_state = 5;
                end

            case 5
                % Release brake
                brake_switch_internal = 1;
                btn_paddle_ri_internal = 1;
                btn_paddle_le_internal = 1;

                main_state = 0;
                sub_state = 0;
        end
end

% Assign outputs from persistent internal values
brake_switch = brake_switch_internal;
btn_paddle_ri = btn_paddle_ri_internal;
btn_paddle_le = btn_paddle_le_internal;

== matlab function GVCU_HIL_simscape/Driver/MATLAB Function1 ==
  settings: updateMethod=DISCRETE
  data: t_sim input; input_mode input; t_pedal input; pedal_data input; acc_pedal_drvr input; brk_pedal_drvr input; t_brake input; pedal_out output; brake_data input; brake_out output
function [pedal_out, brake_out] = fcn(t_sim, input_mode, t_pedal, pedal_data, acc_pedal_drvr, brk_pedal_drvr, t_brake, brake_data)
persistent t_mode_start last_mode;

if isempty(t_mode_start)
    t_mode_start = -1;
    last_mode    = 0;
end

if input_mode == 1 && last_mode ~= 1
    t_mode_start = t_sim;
end
last_mode = input_mode;

if input_mode == 1 && t_mode_start >= 0
    t_rel     = t_sim - t_mode_start;
    pedal_out = interp1(t_pedal, pedal_data, min(t_rel, t_pedal(end)), 'linear', pedal_data(end));
    brake_out = interp1(t_brake, brake_data, min(t_rel, t_brake(end)), 'linear', brake_data(end));
else
    pedal_out = acc_pedal_drvr;
    brake_out = brk_pedal_drvr;
end

== matlab function GVCU_HIL_simscape/Powertrain (EV)/PID Speed Ctrl Mode/MATLAB Function ==
  settings: updateMethod=DISCRETE
  data: EM_Spd input; reset_out output; speed_req input; t input
function reset_out = spdCtrlReset(EM_Spd, speed_req, t)
% Resets PID integrator when both speeds are below threshold for 500ms.
% Matches real inverter: cInvStopSpeed = 20 RPM, SPD_CTRL_RESET_DELAY = 500ms
% Input t: simulation time from Clock block [s]

persistent stop_ts fired

if isempty(stop_ts)
    stop_ts = 0;
    fired   = false;
end

SPD_THRESHOLD  = 2.094;  % 20 RPM in rad/s  (= cInvStopSpeed)
RESET_DELAY_S  = 0.5;    % 500ms in s       (= SPD_CTRL_RESET_DELAY)

if (abs(EM_Spd) < SPD_THRESHOLD) && (abs(speed_req) < SPD_THRESHOLD)
    if stop_ts == 0
        stop_ts = t;     % Start timer: record entry time
    end

    if ((t - stop_ts) >= RESET_DELAY_S) && (~fired)
        reset_out = 1.0; % Rising edge -> reset PID integrator
        fired     = true;
    else
        reset_out = 0.0;
    end
else
    stop_ts   = 0;       % Reset timer
    fired     = false;   % Allow trigger again next standstill
    reset_out = 0.0;
end
